simulink model "invarianza_temporal"  (R2020b)
settings: Solver=VariableStepAuto  StartTime=0.0  StopTime=5  MaxStep=1e-2  RelTol=1e-3
settings Model: Creator=carma  LastModifiedBy=carma
settings DataIOCC: ReturnWorkspaceOutputs=off
settings DebuggingCC: ArithmeticOperatorsInVariantConditions=warning
settings SFSimCC: SimUseLocalCustomCode=off  CustomCodeUndefinedFunction=UseInterfaceOnly
settings RTWCC: RTWUseLocalCustomCode=off

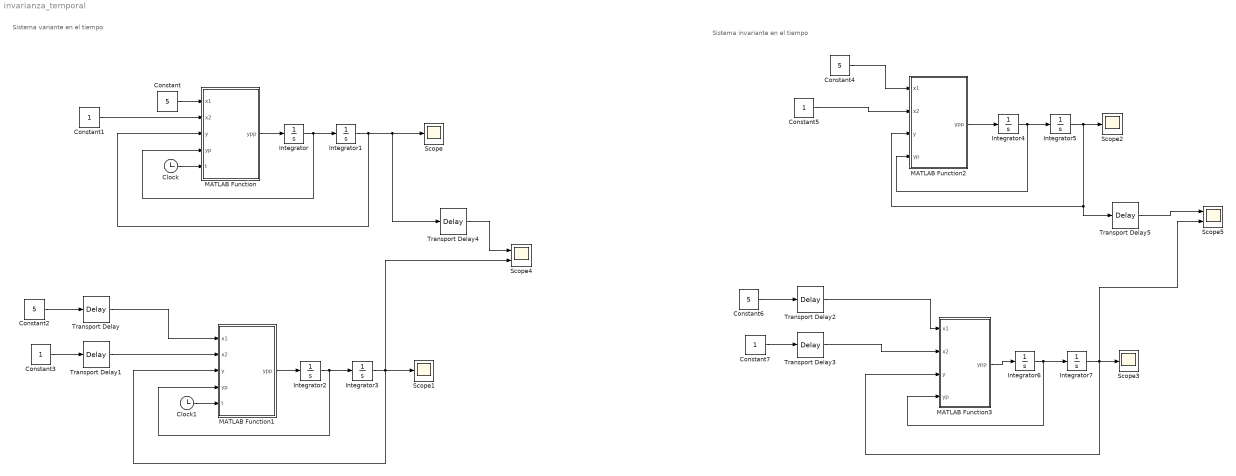
== system invarianza_temporal ==
  note: Sistema variante en el tiempo
  note: Sistema invariante en el tiempo
  Clock : Clock
  Clock1 : Clock
  Constant{,2,4,6} (4 alike) : Constant  Value=5
  Constant{1,3,5,7} (4 alike) : Constant
  Integrator{,1..7} (8 alike) : Integrator
  MATLAB Function : MATLAB Function  TreatAsAtomicUnit=on
  MATLAB Function1 : MATLAB Function  TreatAsAtomicUnit=on
  MATLAB Function2 : MATLAB Function  TreatAsAtomicUnit=on
  MATLAB Function3 : MATLAB Function  TreatAsAtomicUnit=on
  Scope{,1..3} (4 alike) : Scope
  Scope4 : Scope  NumInputPorts=2
  Scope5 : Scope  NumInputPorts=2
  Transport Delay{,1..5} (6 alike) : TransportDelay
  wires:
  MATLAB Function/1(ypp) -> Integrator/1
  Integrator/1 -> Integrator1/1, MATLAB Function/4(yp)
  Integrator1/1 -> MATLAB Function/3(y), Transport Delay4/1, Scope/1
  Clock/1 -> MATLAB Function/5(t)
  Constant/1 -> MATLAB Function/1(x1)
  Constant1/1 -> MATLAB Function/2(x2)
  Integrator3/1 -> Scope4/2, MATLAB Function1/3(y), Scope1/1
  Constant3/1 -> Transport Delay1/1
  Constant2/1 -> Transport Delay/1
  Clock1/1 -> MATLAB Function1/5(t)
  Integrator2/1 -> Integrator3/1, MATLAB Function1/4(yp)
  MATLAB Function1/1(ypp) -> Integrator2/1
  Transport Delay/1 -> MATLAB Function1/1(x1)
  Transport Delay1/1 -> MATLAB Function1/2(x2)
  Transport Delay3/1 -> MATLAB Function3/2(x2)
  Transport Delay2/1 -> MATLAB Function3/1(x1)
  Integrator5/1 -> Transport Delay5/1, MATLAB Function2/3(y), Scope2/1
  Constant4/1 -> MATLAB Function2/1(x1)
  Integrator4/1 -> Integrator5/1, MATLAB Function2/4(yp)
  MATLAB Function2/1(ypp) -> Integrator4/1
  Constant7/1 -> Transport Delay3/1
  Integrator7/1 -> Scope5/2, MATLAB Function3/3(y), Scope3/1
  Integrator6/1 -> MATLAB Function3/4(yp), Integrator7/1
  Constant6/1 -> Transport Delay2/1
  Constant5/1 -> MATLAB Function2/2(x2)
  MATLAB Function3/1(ypp) -> Integrator6/1
  Transport Delay4/1 -> Scope4/1
  Transport Delay5/1 -> Scope5/1

== matlab function invarianza_temporal/MATLAB Function1 ==
  data: x1 input; ypp output; x2 input; y input; yp input; t input
function ypp = fcn(x1,x2,y,yp,t)

ypp =2*x1-6*exp(-2*t)*x2-8*y-4*t*yp;

== matlab function invarianza_temporal/MATLAB Function ==
  data: x1 input; ypp output; x2 input; y input; yp input; t input
function ypp = fcn(x1,x2,y,yp,t)

ypp =2*x1-6*exp(-2*t)*x2-8*y-4*t*yp;

== matlab function invarianza_temporal/MATLAB Function2 ==
  data: x1 input; ypp output; x2 input; y input; yp input
function ypp = fcn(x1,x2,y,yp)

ypp =2*x1-6*x2-8*y-4*yp;

== matlab function invarianza_temporal/MATLAB Function3 ==
  data: x1 input; ypp output; x2 input; y input; yp input
function ypp = fcn(x1,x2,y,yp)

ypp =2*x1-6*x2-8*y-4*yp;
